simulink model "statespace"  (R2016a)
settings: Solver=VariableStepAuto  StartTime=0.0  StopTime=100  RelTol=1e-3
libraries: simulink x1
settings Model: Creator=lm  LastModifiedBy=lm

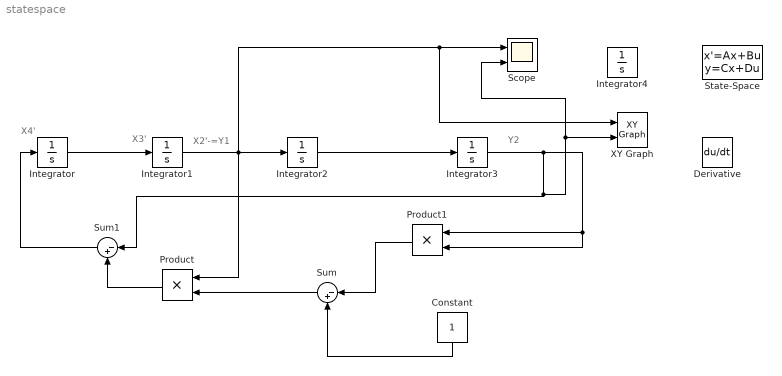
== system statespace ==
  note: Y2
  note: X2'-=Y1
  note: X3'
  note: X4'
  Constant : Constant
  Derivative : Derivative
  Integrator : Integrator
  Integrator1 : Integrator  InitialCondition=0.25
  Integrator2 : Integrator
  Integrator3 : Integrator  InitialCondition=0.25
  Integrator4 : Integrator
  Product : Product
  Product1 : Product
  Scope : Scope  NumInputPorts=2
  State-Space : StateSpace  X0=0
  Sum : Sum  Inputs=|-+
  Sum1 : Sum  Inputs=|-+
  XY Graph : simulink/Sinks/XY Graph  xmin=-1  xmax=1  ymin=-1  ymax=1  st=-1
  wires:
  Integrator/1 -> Integrator1/1
  Integrator1/1 -> XY Graph/1, Scope/1, Product/1, Integrator2/1
  Integrator2/1 -> Integrator3/1
  Integrator3/1 -> Scope/2, XY Graph/2, Sum1/1, Product1/2, Product1/1
  Constant/1 -> Sum/2
  Product1/1 -> Sum/1
  Sum/1 -> Product/2
  Product/1 -> Sum1/2
  Sum1/1 -> Integrator/1
